simulink model "Wawa_Filter_Demo"  (R2019b)
settings: Solver=FixedStepAuto  StartTime=0.0  StopTime=stop_time  FixedStep=mp.Ts_system  RelTol=1e-3
InitFcn:
  | sm_callback_init
StopFcn:
  | sm_callback_stop
values from neighbouring files (symbols this model uses):
  mp = sm_init_avalon_signals(mp)    [sm_callback_init.m]    (also in sm_callback_stop.m = sm_stop_process_output(mp))
libraries: simulink x3, DSP_FPGA_Accelerated_Toolbox x2
settings Model: Creator=Balad  LastModifiedBy=Balad

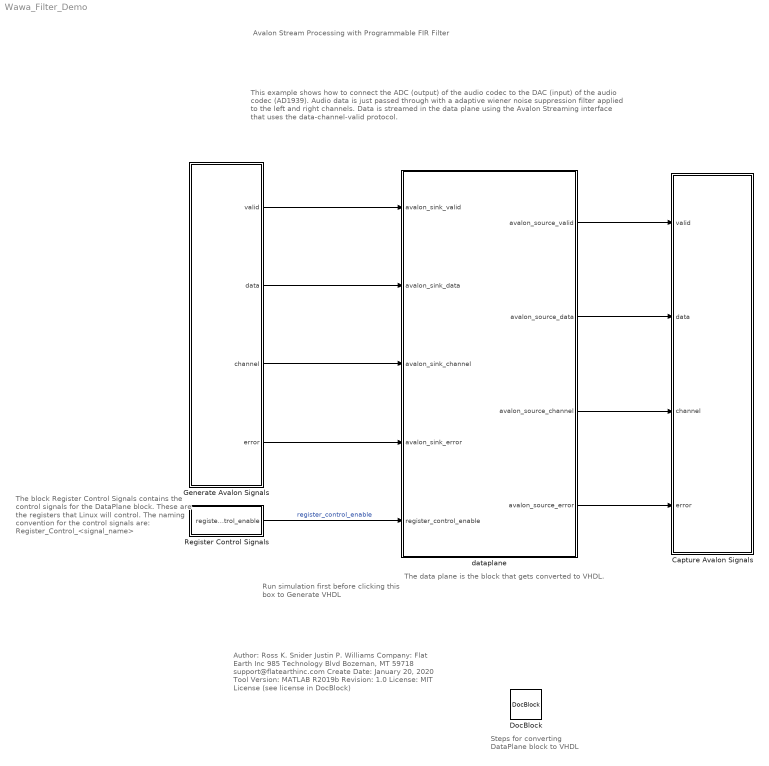
== system Wawa_Filter_Demo ==
  note: Author:          Ross K. Snider
      |                      Justin P. Williams
      | Company:     Flat Earth Inc
      |                       985 Technology Blvd
      |                       Bozeman, MT 59718
      |                       support@flatearthinc.com
      | Create Date:  January 20, 2020
      | Tool Version:  MATLAB R2019b
      | Revision:        1.0
      | License:          MIT License (see license in DocBlock)
  note: The data plane is the block that gets converted to VHDL.
  note: Steps for converting
      | DataPlane block
      | to VHDL
  note: Avalon Stream Processing
      | with Programmable FIR Filter
  note: Run simulation first
      | before clicking this box to
      | Generate VHDL
  note: This example shows how to connect the ADC (output) of the audio codec to the DAC (input) of the audio codec (AD1939). Audio data is just passed through with a adaptive wiener noise suppression filter applied to the left and right channels. Data is streamed in the data plane using the Avalon Streaming interface that uses the data-channel-valid protocol.
  note: The block Register Control Signals contains
      | the control signals for the DataPlane block.
      | These are the registers that Linux will control.
      | The naming convention for the control
      | signals are:  Register_Control_<signal_name>
  Capture Avalon Signals : Subsystem
  DocBlock : simulink/Model-Wide Utilities/DocBlock  DocumentType=HTML
  Generate Avalon Signals : Subsystem
  Register Control Signals : Subsystem
  dataplane : Subsystem  TreatAsAtomicUnit=on
  wires:
  dataplane/4(avalon_source_error) -> Capture Avalon Signals/4(error)
  Register Control Signals/1(register_control_enable) -> dataplane/5(register_control_enable)  "register_control_enable"
  Generate Avalon Signals/2(data) -> dataplane/2(avalon_sink_data)
  Generate Avalon Signals/4(error) -> dataplane/4(avalon_sink_error)
  Generate Avalon Signals/3(channel) -> dataplane/3(avalon_sink_channel)
  Generate Avalon Signals/1(valid) -> dataplane/1(avalon_sink_valid)
  dataplane/3(avalon_source_channel) -> Capture Avalon Signals/3(channel)
  dataplane/1(avalon_source_valid) -> Capture Avalon Signals/1(valid)
  dataplane/2(avalon_source_data) -> Capture Avalon Signals/2(data)

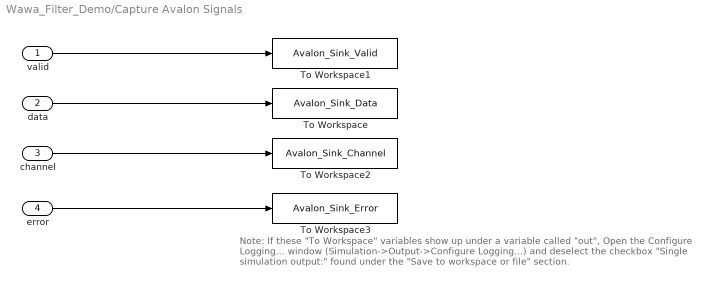
== system Wawa_Filter_Demo/Capture Avalon Signals ==
  note: Note:  If these "To Workspace" variables show up under a variable called "out",
      | Open the Configure Logging... window (Simulation->Output->Configure Logging...)
      | and deselect the checkbox "Single simulation output:" found under the "Save to workspace or file" section.
  valid : Inport
  data : Inport  Port=2
  channel : Inport  Port=3
  error : Inport  Port=4
  To Workspace : ToWorkspace  VariableName=Avalon_Sink_Data  SaveFormat=Timeseries  SampleTime=-1
  To Workspace1 : ToWorkspace  VariableName=Avalon_Sink_Valid  SaveFormat=Timeseries  SampleTime=-1
  To Workspace2 : ToWorkspace  VariableName=Avalon_Sink_Channel  SaveFormat=Timeseries  SampleTime=-1
  To Workspace3 : ToWorkspace  VariableName=Avalon_Sink_Error  SaveFormat=Timeseries  SampleTime=-1
  wires:
  data/1 -> To Workspace/1
  valid/1 -> To Workspace1/1
  error/1 -> To Workspace3/1
  channel/1 -> To Workspace2/1

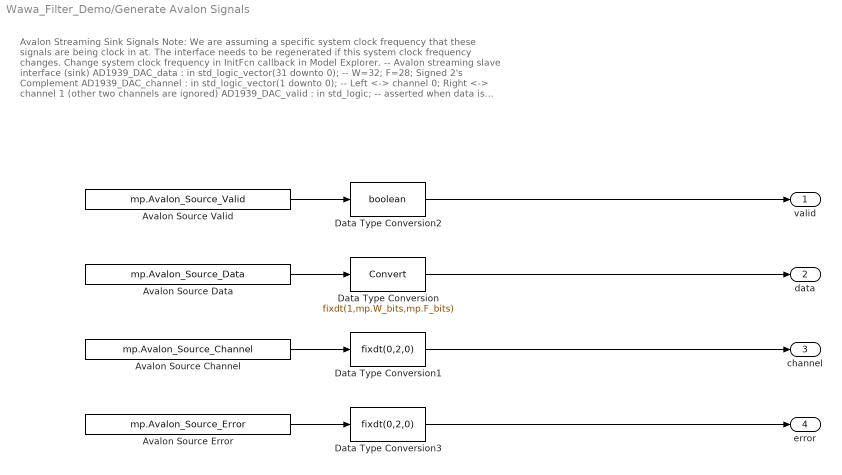
== system Wawa_Filter_Demo/Generate Avalon Signals ==
  note: Avalon Streaming Sink Signals
      | Note: We are assuming a specific system clock frequency that these signals are being clock in at.
      | The interface needs to be regenerated if this system clock frequency changes. Change system clock frequency in InitFcn callback in Model Explorer.
      |
      | -- Avalon streaming slave interface (sink)
      | AD1939_DAC_data : in std_logic_vector(31 downto 0); -- W=32; F=28; Signed 2's Complement
      | AD1939_DAC_channel : in std_logic_vector(1 downto 0); -- Left <-> channel 0; Right <-> channel 1 (other two channels are ignored)
      | AD1939_DAC_valid : in std_logic; -- asserted when data is valid
      | AD1939_DAC_error : in std_logic_vector(1 downto 0) -- error channel is ignored, assumed to be error free at this point
      |
      | For more information on the data-channel-valid protocol, s ee chapter 5 in Intel's Avalon Interfaced Specification (p. 40) at https://www.intel.com/content/dam/www/programmable/us/en/pdfs/literature/manual/mnl_avalon_spec.pdf
  Avalon Source Channel : FromWorkspace  VariableName=mp.Avalon_Source_Channel  OutDataTypeStr=double  SampleTime=mp.Ts_system
  "Avalon Source Data " : FromWorkspace  VariableName=mp.Avalon_Source_Data  OutDataTypeStr=double  SampleTime=mp.Ts_system
  Avalon Source Error : FromWorkspace  VariableName=mp.Avalon_Source_Error  OutDataTypeStr=double  SampleTime=mp.Ts_system
  Avalon Source Valid : FromWorkspace  VariableName=mp.Avalon_Source_Valid  OutDataTypeStr=double  SampleTime=mp.Ts_system
  Data Type Conversion : DataTypeConversion  OutDataTypeStr=fixdt(1,mp.W_bits,mp.F_bits)
  Data Type Conversion1 : DataTypeConversion  OutDataTypeStr=fixdt(0,2,0)
  Data Type Conversion2 : DataTypeConversion  OutDataTypeStr=boolean
  Data Type Conversion3 : DataTypeConversion  OutDataTypeStr=fixdt(0,2,0)
  valid : Outport  VectorParamsAs1DForOutWhenUnconnected=off
  data : Outport  Port=2  VectorParamsAs1DForOutWhenUnconnected=off
  channel : Outport  Port=3  VectorParamsAs1DForOutWhenUnconnected=off
  error : Outport  Port=4  VectorParamsAs1DForOutWhenUnconnected=off
  wires:
  Data Type Conversion1/1 -> channel/1
  Data Type Conversion2/1 -> valid/1
  Avalon Source Error/1 -> Data Type Conversion3/1
  Data Type Conversion/1 -> data/1
  Avalon Source Valid/1 -> Data Type Conversion2/1
  Data Type Conversion3/1 -> error/1
  Avalon Source Channel/1 -> Data Type Conversion1/1
  "Avalon Source Data "/1 -> Data Type Conversion/1

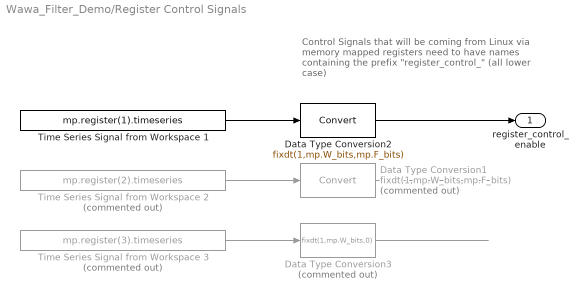
== system Wawa_Filter_Demo/Register Control Signals ==
  note: Control Signals that will be coming from Linux via
      | memory mapped registers need to have names
      | containing the prefix "register_control_"
      | (all lower case)
  Data Type Conversion1 : DataTypeConversion  Commented=on  OutDataTypeStr=fixdt(1,mp.W_bits,mp.F_bits)
  Data Type Conversion2 : DataTypeConversion  OutDataTypeStr=fixdt(1,mp.W_bits,mp.F_bits)
  Data Type Conversion3 : DataTypeConversion  Commented=on  OutDataTypeStr=fixdt(1,mp.W_bits,0)
  Time Series Signal from Workspace 1 : FromWorkspace  VariableName=mp.register(1).timeseries  OutDataTypeStr=double  SampleTime=mp.Ts_system
  Time Series Signal from Workspace 2 : FromWorkspace  Commented=on  VariableName=mp.register(2).timeseries  OutDataTypeStr=double  SampleTime=mp.Ts_system
  Time Series Signal from Workspace 3 : FromWorkspace  Commented=on  VariableName=mp.register(3).timeseries  OutDataTypeStr=double  SampleTime=mp.Ts_system
  register_control_enable : Outport  VectorParamsAs1DForOutWhenUnconnected=off
  wires:
  Time Series Signal from Workspace 2/1 -> Data Type Conversion1/1
  Time Series Signal from Workspace 1/1 -> Data Type Conversion2/1
  Data Type Conversion2/1 -> register_control_enable/1
  Data Type Conversion1/1 -> ?
  Time Series Signal from Workspace 3/1 -> Data Type Conversion3/1
  Data Type Conversion3/1 -> ?

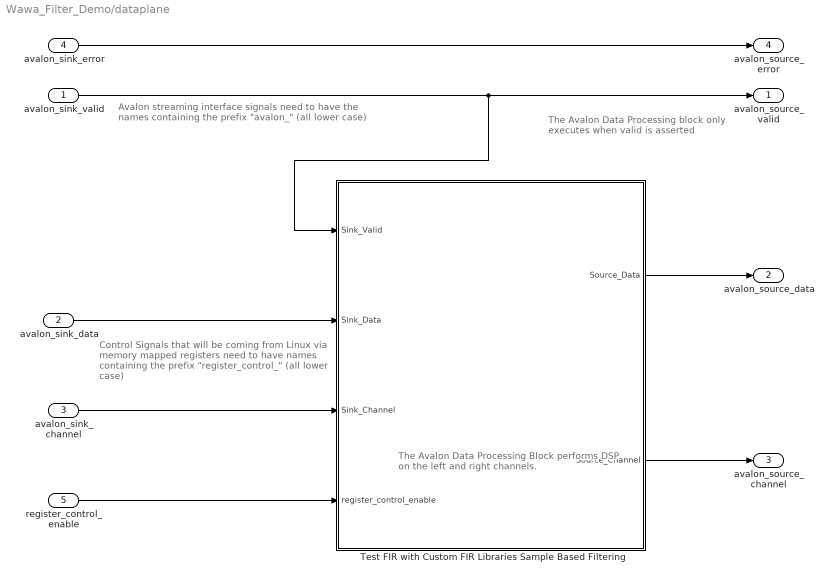
== system Wawa_Filter_Demo/dataplane ==
  note: Control Signals that will be coming from Linux via
      | memory mapped registers need to have names
      | containing the prefix "register_control_"
      | (all lower case)
  note: The Avalon Data Processing Block
      | performs DSP on the left and right channels.
  note: The Avalon Data Processing block
      | only executes when valid is asserted
  note: Avalon streaming interface signals need to have the
      | names containing the prefix "avalon_"
      | (all lower case)
  avalon_sink_valid : Inport
  avalon_sink_data : Inport  Port=2
  avalon_sink_channel : Inport  Port=3
  avalon_sink_error : Inport  Port=4
  register_control_enable : Inport  Port=5
  Test FIR with Custom FIR Libraries Sample Based Filtering : Subsystem
  avalon_source_valid : Outport  VectorParamsAs1DForOutWhenUnconnected=off
  avalon_source_data : Outport  Port=2  VectorParamsAs1DForOutWhenUnconnected=off
  avalon_source_channel : Outport  Port=3  VectorParamsAs1DForOutWhenUnconnected=off
  avalon_source_error : Outport  Port=4  VectorParamsAs1DForOutWhenUnconnected=off
  wires:
  avalon_sink_error/1 -> avalon_source_error/1
  Test FIR with Custom FIR Libraries Sample Based Filtering/1(Source_Data) -> avalon_source_data/1
  avalon_sink_valid/1 -> Test FIR with Custom FIR Libraries Sample Based Filtering/1(Sink_Valid), avalon_source_valid/1
  avalon_sink_data/1 -> Test FIR with Custom FIR Libraries Sample Based Filtering/2(Sink_Data)
  Test FIR with Custom FIR Libraries Sample Based Filtering/2(Source_Channel) -> avalon_source_channel/1
  avalon_sink_channel/1 -> Test FIR with Custom FIR Libraries Sample Based Filtering/3(Sink_Channel)
  register_control_enable/1 -> Test FIR with Custom FIR Libraries Sample Based Filtering/4(register_control_enable)

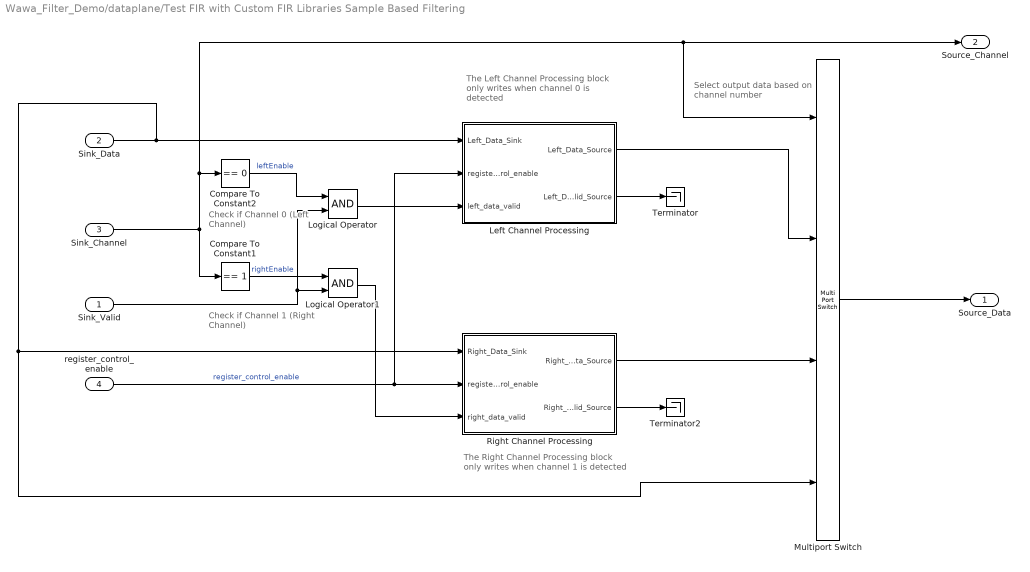
== system Wawa_Filter_Demo/dataplane/Test FIR with Custom FIR Libraries Sample Based Filtering ==
  note: The Left Channel Processing block
      | only writes when channel 0
      | is detected
  note: The Right Channel Processing block
      | only writes when channel 1
      | is detected
  note: Check if Channel 0
      | (Left Channel)
  note: Select output data
      | based on channel number
  note: Check if Channel 1
      | (Right Channel)
  Sink_Valid : Inport
  Sink_Data : Inport  Port=2
  Sink_Channel : Inport  Port=3
  register_control_enable : Inport  Port=4
  Compare To Constant1 : simulink/Logic and Bit Operations/Compare To Constant  relop===  const=1  OutDataTypeStr=boolean
  Compare To Constant2 : simulink/Logic and Bit Operations/Compare To Constant  relop===  const=0  OutDataTypeStr=boolean
  Left Channel Processing : Subsystem  TreatAsAtomicUnit=on
  Logical Operator : Logic  AllPortsSameDT=off  OutDataTypeStr=boolean
  Logical Operator1 : Logic  AllPortsSameDT=off  OutDataTypeStr=boolean
  Multiport Switch : MultiPortSwitch  DataPortOrder=Zero-based contiguous  DiagnosticForDefault=None  zeroidx=on
  Right Channel Processing : Subsystem  TreatAsAtomicUnit=on
  Terminator : Terminator
  Terminator2 : Terminator
  Source_Data : Outport  InitialOutput=0  VectorParamsAs1DForOutWhenUnconnected=off
  Source_Channel : Outport  Port=2  InitialOutput=0  VectorParamsAs1DForOutWhenUnconnected=off
  wires:
  Left Channel Processing/1("Left_Data_Source ") -> Multiport Switch/2
  Multiport Switch/1 -> Source_Data/1
  Compare To Constant2/1 -> Logical Operator/1  "leftEnable"
  Sink_Data/1 -> Multiport Switch/4, Right Channel Processing/1(Right_Data_Sink), Left Channel Processing/1(Left_Data_Sink)
  Right Channel Processing/1("Right_Data_Source ") -> Multiport Switch/3
  Sink_Channel/1 -> Source_Channel/1, Multiport Switch/1, Compare To Constant2/1, Compare To Constant1/1
  Compare To Constant1/1 -> Logical Operator1/1  "rightEnable"
  register_control_enable/1 -> Left Channel Processing/2(register_control_enable), Right Channel Processing/2(register_control_enable)  "register_control_enable"
  Left Channel Processing/2(Left_Data_Valid_Source) -> Terminator/1
  Right Channel Processing/2(Right_Data_Valid_Source) -> Terminator2/1
  Sink_Valid/1 -> Logical Operator/2, Logical Operator1/2
  Logical Operator/1 -> Left Channel Processing/3(left_data_valid)
  Logical Operator1/1 -> Right Channel Processing/3(right_data_valid)

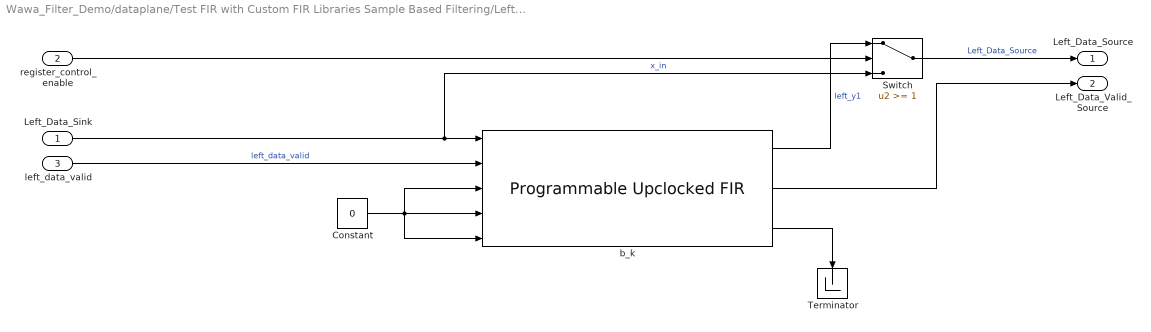
== system Wawa_Filter_Demo/dataplane/Test FIR with Custom FIR Libraries Sample Based Filtering/Left Channel Processing ==
  Left_Data_Sink : Inport
  register_control_enable : Inport  Port=2
  left_data_valid : Inport  Port=3
  Constant : Constant  Value=0  SampleTime=-1
  Switch : Switch  Threshold=1
  Terminator : Terminator
  b_k : DSP_FPGA_Accelerated_Toolbox/Programmable Upclocked FIR  b_k=lpFiltFi  Ts=1/48000  rotationDelay=0  W_bits=32  F_bits=28
  "Left_Data_Source " : Outport  InitialOutput=0  VectorParamsAs1DForOutWhenUnconnected=off
  Left_Data_Valid_Source : Outport  Port=2  InitialOutput=0  VectorParamsAs1DForOutWhenUnconnected=off
  wires:
  register_control_enable/1 -> Switch/2
  Left_Data_Sink/1 -> Switch/3, b_k/1  "x_in"
  Switch/1 -> "Left_Data_Source "/1  "Left_Data_Source"
  left_data_valid/1 -> b_k/2  "left_data_valid"
  Constant/1 -> b_k/5, b_k/3, b_k/4
  b_k/3 -> Terminator/1
  b_k/1 -> Switch/1  "left_y1"
  b_k/2 -> Left_Data_Valid_Source/1

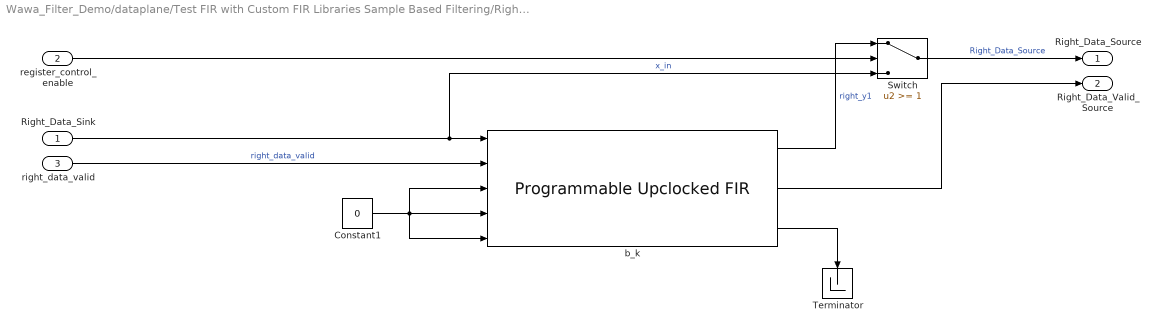
== system Wawa_Filter_Demo/dataplane/Test FIR with Custom FIR Libraries Sample Based Filtering/Right Channel Processing ==
  Right_Data_Sink : Inport
  register_control_enable : Inport  Port=2
  right_data_valid : Inport  Port=3
  Constant1 : Constant  Value=0  SampleTime=-1
  Switch : Switch  Threshold=1
  Terminator : Terminator
  b_k : DSP_FPGA_Accelerated_Toolbox/Programmable Upclocked FIR  b_k=lpFiltFi  Ts=1/48000  rotationDelay=0  W_bits=32  F_bits=28
  "Right_Data_Source " : Outport  InitialOutput=0  VectorParamsAs1DForOutWhenUnconnected=off
  Right_Data_Valid_Source : Outport  Port=2  InitialOutput=0  VectorParamsAs1DForOutWhenUnconnected=off
  wires:
  Switch/1 -> "Right_Data_Source "/1  "Right_Data_Source"
  b_k/3 -> Terminator/1
  Right_Data_Sink/1 -> Switch/3, b_k/1  "x_in"
  right_data_valid/1 -> b_k/2  "right_data_valid"
  Constant1/1 -> b_k/5, b_k/3, b_k/4
  register_control_enable/1 -> Switch/2
  b_k/1 -> Switch/1  "right_y1"
  b_k/2 -> Right_Data_Valid_Source/1
